simulink model "GREEN_CARM_DARM"  (Simulink 9.0)
settings: Solver=ode45  StartTime=0.0  StopTime=10.0  RelTol=1e-3  AbsTol=1e-6
values from neighbouring files (symbols this model uses):
  Actuator = [1,1/2;1,-1/2]    [run_NBGREEN_CARM_DARM.m]
  Changing_unit1 = c/L/532e-9    (= 187839885965)    [run_NBGREEN_CARM_DARM.m]
  CMRR_arm = 1    [run_NBGREEN_CARM_DARM.m]
  Noise = containers.Map    [run_NBGREEN_CARM_DARM.m]
  Sensing = [1,0;0,-1]    [run_NBGREEN_CARM_DARM.m]
  TransImp = containers.Map    [run_NBGREEN_CARM_DARM.m]
  use_AOM = 1    [run_NBGREEN_CARM_DARM.m]
  VertCoup = 0.01    [run_NBGREEN_CARM_DARM.m]
undefined symbols (not defined in the file or in its folder): Act, Cav, CavOpgain, CMS_SW_IMC, dt, myzpk, Suspension, SW
libraries: cstblocks x42, NbLibrary x35, mnNb_Lib x5
CloseFcn:
  | ;slview('closediagram',bdroot);
settings Model: SuppressorTable=22 serialization::archive 11 0 6 0 0 0 0 0  Creator=controls  LastModifiedBy=miyo  ExtModeTrigMode=oneshot  ExtModeArmWhenConnect=off
settings DataIOCC: SignalLoggingSaveFormat=ModelDataLogs
settings OptimizationCC: BlockReduction=off  BooleanDataType=off  DefaultParameterBehavior=Inlined  BufferReuse=off
settings DebuggingCC: SaveWithParameterizedLinksMsg=none  SignalResolutionControl=TryResolveAllWithWarning  MultiTaskDSMMsg=warning  MultiTaskCondExecSysMsg=none  StateNameClashWarn=warning  InitInArrayFormatMsg=none
settings HardwareCC: TargetUnknown=on
settings RTWCC: TemplateMakefile=grt_unix.tmf
settings GRTTargetCC: GeneratePreprocessorConditionals=Disable all  CombineOutputUpdateFcns=off  GRTInterface=on
settings ConfigComp: CovSFcnEnable=off

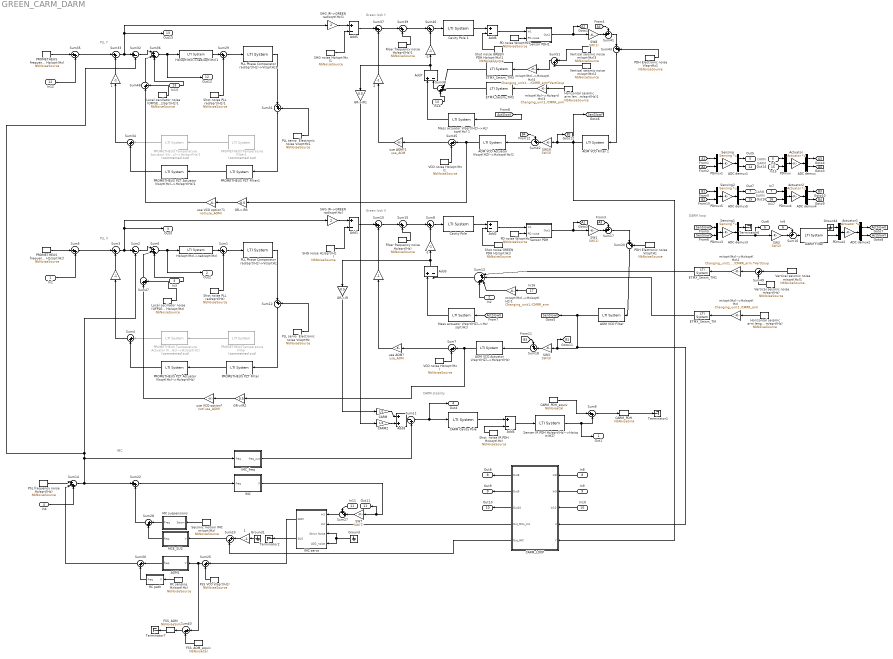
== system GREEN_CARM_DARM ==
  note: PLL X
  note: Green lock X
  note: IMC
  note: CARM stablity
  note: PLL Y
  note: Green lock Y
  note: CARM
  note: DARM
  note: CARM
  note: DARM
  note: DARM loop
  In1 : Inport
  In2 : Inport  Port=2
  In3 : Inport  Port=3
  In4 : Inport  Port=4
  In5 : Inport  Port=5
  In6 : Inport  Port=6
  In7 : Inport  Port=7
  In8 : Inport  Port=8
  In9 : Inport  Port=9
  In10 : Inport  Port=10
  In11 : Inport  Port=11
  In12 : Inport  Port=12
  In13 : Inport  Port=13
  In14 : Inport  Port=14
  In15 : Inport  Port=15
  In17 : Inport  Port=16
  In16 : Inport  Port=17
  " " : Gain  Gain=-1
  "  " : Gain  Gain=-1
  "  1" : Gain  Gain=-1
  " -1" : Gain  Gain=-1
  " -2" : Gain  Gain=-1
  " 1" : Gain  Gain=-1
  " 2" : Gain  Gain=-1
   GR->IR{,1..3} (4 alike) : Gain  Gain=0.5
  ADC demux{,1..5} (6 alike) : Demux  Outputs=2
  AOM VCO Actuator V/sqrt(HZ)-->Hz/sqrt(Hz) : cstblocks/LTI System  sys=Act_AOM_X  IC=[]
  AOM VCO Actuator V/sqrt(HZ)-->Hz/sqrt(Hz)1 : cstblocks/LTI System  sys=Act_AOM_Y  IC=[]
  "AOM VCO Filter " : cstblocks/LTI System  sys=Filt_GR1  IC=[]
  AOM VCO Filter 1 : cstblocks/LTI System  sys=Filt_GR1  IC=[]
  AOM1 : Subsystem
  Actuator : Gain  Gain=Actuator  Multiplication=Matrix(K*u)
  Actuator1 : Gain  Gain=Actuator  Multiplication=Matrix(K*u)
  Actuator2 : Gain  Gain=Actuator  Multiplication=Matrix(K*u)
  Add{1..7} (7 alike) : Sum  Inputs=+-
  Add8 : Sum
  CARM : Gain  Gain=1/2
  CARM Cavity Pole : cstblocks/LTI System  sys=CARM_Cavity_Pole  IC=[]
  CARM2 : Gain  Gain=1/2
  CARM_LOOP : Subsystem
  CARM_PDH : NbLibrary/NbNoiseSink  Tag=NbNoiseSink  dof='CARM'  asd=''  chan=''
      settings: AttributesFormatString=%<Tag>
  CARM_PDH_equiv : NbLibrary/NbNoiseCal  Tag=NbNoiseCal  dof='CARM'  unit='Frequency noise [Hz/rtHz]'
      settings: AttributesFormatString=%<Tag>
  "Cavity Pole " : cstblocks/LTI System  sys=Cavity_Pole  IC=[]
  Cavity Pole 1 : cstblocks/LTI System  sys=Cavity_Pole  IC=[]
  "DARM Filter " : cstblocks/LTI System  sys=Filt_darm  IC=[]
  ETMX_Seism_TM : cstblocks/LTI System  Description=FlexTf: Susp('ETMX_Seism_TM')  sys=1  IC=[]
      settings: AttributesFormatString=%<Description>
  ETMX_Seism_TM1 : cstblocks/LTI System  Description=FlexTf: Susp('ETMX_Seism_Vert')  sys=1  IC=[]
      settings: AttributesFormatString=%<Description>
  ETMX_Seism_TM2 : cstblocks/LTI System  Description=FlexTf: Susp('ETMX_Seism_TM')  sys=1  IC=[]
      settings: AttributesFormatString=%<Description>
  ETMX_Seism_TM3 : cstblocks/LTI System  Description=FlexTf: Susp('ETMX_Seism_Vert')  sys=1  IC=[]
      settings: AttributesFormatString=%<Description>
  FSS VCO V/sqrt(Hz) : NbLibrary/NbNoiseSource  Tag=NbNoiseSource  asd=Noise('act_AOM')  chan=''  groupNest=1  group='IR noise'  subgroup=''  subsubgroup=''  subsubsubgroup=''
      settings: AttributesFormatString=%<Tag>
  FSS_AOM : NbLibrary/NbNoiseSink  Tag=NbNoiseSink  dof='FSS_AOM'  asd=''  chan=''
      settings: AttributesFormatString=%<Tag>
  FSS_AOM_equiv : NbLibrary/NbNoiseCal  Tag=NbNoiseCal  dof='FSS_AOM'  unit='Feedback signal [V/rtHz]'
      settings: AttributesFormatString=%<Tag>
  Fiber frequency noise Hz/sqrt(Hz) : NbLibrary/NbNoiseSource  Tag=NbNoiseSource  asd=Noise('Fiber')  chan=''  groupNest=1  group='Green noise'  subgroup=''  subsubgroup=''  subsubsubgroup=''
      settings: AttributesFormatString=%<Tag>
  Fiber frequency noise Hz/sqrt(Hz)1 : NbLibrary/NbNoiseSource  Tag=NbNoiseSource  asd=Noise('Fiber')  chan=''  groupNest=1  group='Green noise'  subgroup=''  subsubgroup=''  subsubsubgroup=''
      settings: AttributesFormatString=%<Tag>
  Ground : Ground
  Ground1 : Ground
  Ground4 : Ground
  Horizontal seismic arm length m/sqrt(Hz) : NbLibrary/NbNoiseSource  Tag=NbNoiseSource  asd=Noise('Seismic arm length')  chan=''  groupNest=1  group='Seismic noise'  subgroup=''  subsubgroup=''  subsubsubgroup=''
      settings: AttributesFormatString=%<Tag>
  Horizontal seismic arm length m/sqrt(Hz)1 : NbLibrary/NbNoiseSource  Tag=NbNoiseSource  asd=Noise('Seismic arm length')  chan=''  groupNest=1  group='Seismic noise'  subgroup=''  subsubgroup=''  subsubsubgroup=''
      settings: AttributesFormatString=%<Tag>
  Hz/sqrt(Hz)->rad/sqrt(Hz) : cstblocks/LTI System  sys=Changing_unit  IC=[]
  Hz/sqrt(Hz)->rad/sqrt(Hz)1 : cstblocks/LTI System  sys=Changing_unit  IC=[]
  IMC : Subsystem
  IMC servo : Subsystem
  IMC_freq : Subsystem
  Local oscillator noise (OFFSET) Hz/sqrt(Hz) : NbLibrary/NbNoiseSource  Tag=NbNoiseSource  asd=Noise('LO noise')  chan=''  groupNest=1  group='PLL noise'  subgroup=''  subsubgroup=''  subsubsubgroup=''
      settings: AttributesFormatString=%<Tag>
  Local oscillator noise (OFFSET) Hz/sqrt(Hz)1 : NbLibrary/NbNoiseSource  Tag=NbNoiseSource  asd=Noise('LO noise')  chan=''  groupNest=1  group='PLL noise'  subgroup=''  subsubgroup=''  subsubsubgroup=''
      settings: AttributesFormatString=%<Tag>
  MC suspensions : Subsystem
  MCE_SUS : Subsystem
  "Mass actuator V/sqrt(HZ)-->Hz/sqrt(Hz) " : cstblocks/LTI System  sys=Act_mass  IC=[]
  Mass actuator V/sqrt(HZ)-->Hz/sqrt(Hz) 1 : cstblocks/LTI System  sys=Act_mass  IC=[]
  PD noise W/sqrtHz : NbLibrary/NbNoiseSource  Tag=NbNoiseSource  asd=Noise('PD noise PDH')  chan=''  groupNest=1  group='Green noise'  subgroup=''  subsubgroup=''  subsubsubgroup=''
      settings: AttributesFormatString=%<Tag>
  PD noise W/sqrtHz1 : NbLibrary/NbNoiseSource  Tag=NbNoiseSource  asd=Noise('PD noise PDH')  chan=''  groupNest=1  group='Green noise'  subgroup=''  subsubgroup=''  subsubsubgroup=''
      settings: AttributesFormatString=%<Tag>
  PDH Electronic noise V/sqrtHz : NbLibrary/NbNoiseSource  Tag=NbNoiseSource  asd=Noise('Electronic noise PDH')  chan=''  groupNest=1  group='Green noise'  subgroup=''  subsubgroup=''  subsubsubgroup=''
      settings: AttributesFormatString=%<Tag>
  PDH Electronic noise V/sqrtHz1 : NbLibrary/NbNoiseSource  Tag=NbNoiseSource  asd=Noise('Electronic noise PDH')  chan=''  groupNest=1  group='Green noise'  subgroup=''  subsubgroup=''  subsubsubgroup=''
      settings: AttributesFormatString=%<Tag>
  PDmux{,1..5} (6 alike) : Mux  Inputs=2
  PLL Phase Comparator rad/sqrt(Hz)->V/sqrtHz : cstblocks/LTI System  sys=Sen  IC=[]
  PLL Phase Comparator rad/sqrt(Hz)->V/sqrtHz1 : cstblocks/LTI System  sys=Sen  IC=[]
  PLL servo  Electronic noise V/sqrtHz : NbLibrary/NbNoiseSource  Tag=NbNoiseSource  asd=Noise('Electronic noise PLL')  chan=''  groupNest=1  group='PLL noise'  subgroup=''  subsubgroup=''  subsubsubgroup=''
      settings: AttributesFormatString=%<Tag>
  PLL servo  Electronic noise V/sqrtHz1 : NbLibrary/NbNoiseSource  Tag=NbNoiseSource  asd=Noise('Electronic noise PLL')  chan=''  groupNest=1  group='PLL noise'  subgroup=''  subsubgroup=''  subsubsubgroup=''
      settings: AttributesFormatString=%<Tag>
  PROMETHEUS PZT Actuator V/sqrt(Hz)-->Hz/sqrt(Hz) : cstblocks/LTI System  sys=Act_PZT  IC=[]
  PROMETHEUS PZT Actuator V/sqrt(Hz)-->Hz/sqrt(Hz)1 : cstblocks/LTI System  sys=Act_PZT  IC=[]
  PROMETHEUS PZT Filter : cstblocks/LTI System  sys=Filt_PZT  IC=[]
  PROMETHEUS PZT Filter1 : cstblocks/LTI System  sys=Filt_PZT  IC=[]
  PROMETHEUS Temperature Actuator V/sqrt(Hz)-->Hz/sqrt(Hz) : cstblocks/LTI System  Commented=on  sys=Act_Temp  IC=[]
  PROMETHEUS Temperature Actuator V/sqrt(Hz)-->Hz/sqrt(Hz)1 : cstblocks/LTI System  Commented=on  sys=Act_Temp  IC=[]
  PROMETHEUS frequency noise X Hz/sqrt(Hz) : NbLibrary/NbNoiseSource  Tag=NbNoiseSource  asd=Noise('Prometheus freq noise')  chan=''  groupNest=1  group='PLL noise'  subgroup=''  subsubgroup=''  subsubsubgroup=''
      settings: AttributesFormatString=%<Tag>
  PROMETHEUS frequency noise Y Hz/sqrt(Hz) : NbLibrary/NbNoiseSource  Tag=NbNoiseSource  asd=Noise('Prometheus freq noise')  chan=''  groupNest=1  group='PLL noise'  subgroup=''  subsubgroup=''  subsubsubgroup=''
      settings: AttributesFormatString=%<Tag>
  PROMETHEUSTemperature Filter : cstblocks/LTI System  Commented=on  sys=Filt_Temp  IC=[]
  PROMETHEUSTemperature Filter1 : cstblocks/LTI System  Commented=on  sys=Filt_Temp  IC=[]
  PSL frequency noise Hz/sqrt(Hz) : NbLibrary/NbNoiseSource  Tag=NbNoiseSource  asd=Noise('PSL freq noise')*0  chan=''  groupNest=1  group='IR noise'  subgroup=''  subsubgroup=''  subsubsubgroup=''
      settings: AttributesFormatString=%<Tag>
  RC path : Subsystem
  RC sensing Hz/sqrt(Hz) : NbLibrary/NbNoiseSource  Tag=NbNoiseSource  asd=Noise('sensor_RefCav')  chan=''  groupNest=1  group='IR noise'  subgroup=''  subsubgroup=''  subsubsubgroup=''
      settings: AttributesFormatString=%<Tag>
  SHG IR-->GREEN rad/sqrt(Hz) : Gain  Gain=2
  SHG IR-->GREEN rad/sqrt(Hz)1 : Gain  Gain=2
  SHG noise Hz/sqrt(Hz) : NbLibrary/NbNoiseSource  Tag=NbNoiseSource  asd=Noise('SHG')  chan=''  groupNest=1  group='Green noise'  subgroup=''  subsubgroup=''  subsubsubgroup=''
      settings: AttributesFormatString=%<Tag>
  SHG noise Hz/sqrt(Hz)1 : NbLibrary/NbNoiseSource  Tag=NbNoiseSource  asd=Noise('SHG')  chan=''  groupNest=1  group='Green noise'  subgroup=''  subsubgroup=''  subsubsubgroup=''
      settings: AttributesFormatString=%<Tag>
  SW1 : Gain  Gain=SW(1)
  SW10 : Gain  Gain=SW(3)
  SW2 : Gain  Gain=SW(2)
  SW3 : Gain  Gain=SW(3)
  SW7 : Gain  Gain=SW(7)
  SW8 : Gain  Gain=SW(1)
  Seismic motion IMC m/sqrt(Hz) : NbLibrary/NbNoiseSource  Tag=NbNoiseSource  asd=Noise('seismic_IMC')  chan=''  groupNest=1  group='IR noise'  subgroup=''  subsubgroup=''  subsubsubgroup=''
      settings: AttributesFormatString=%<Tag>
  Senser IR PDH Hz/sqrt(Hz)-->Hz/sqrt(HZ) : cstblocks/LTI System  sys=Sen_2  IC=[]
  Sensing : Gain  Gain=Sensing  Multiplication=Matrix(K*u)
  Sensing1 : Gain  Gain=Sensing  Multiplication=Matrix(K*u)
  Sensing2 : Gain  Gain=Sensing  Multiplication=Matrix(K*u)
  Sensor PDH : Subsystem
  Sensor PDH1 : Subsystem
  Shot  noise IR PDH Hz/sqrt(Hz) : NbLibrary/NbNoiseSource  Tag=NbNoiseSource  asd=Noise('Shot noise IR')  chan=''  groupNest=1  group='IR noise'  subgroup=''  subsubgroup=''  subsubsubgroup=''
      settings: AttributesFormatString=%<Tag>
  Shot noise GREEN PDH Hz/sqrt(Hz) : NbLibrary/NbNoiseSource  Tag=NbNoiseSource  asd=Noise('Shot noise green')  chan=''  groupNest=1  group='Green noise'  subgroup=''  subsubgroup=''  subsubsubgroup=''
      settings: AttributesFormatString=%<Tag>
  Shot noise GREEN PDH Hz/sqrt(Hz)1 : NbLibrary/NbNoiseSource  Tag=NbNoiseSource  asd=Noise('Shot noise green')  chan=''  groupNest=1  group='Green noise'  subgroup=''  subsubgroup=''  subsubsubgroup=''
      settings: AttributesFormatString=%<Tag>
  Shot noise PLL rad/sqrt(Hz) : NbLibrary/NbNoiseSource  Tag=NbNoiseSource  asd=Noise('Shot noise PLL')  chan=''  groupNest=1  group='PLL noise'  subgroup=''  subsubgroup=''  subsubsubgroup=''
      settings: AttributesFormatString=%<Tag>
  Shot noise PLL rad/sqrt(Hz)1 : NbLibrary/NbNoiseSource  Tag=NbNoiseSource  asd=Noise('Shot noise PLL')  chan=''  groupNest=1  group='PLL noise'  subgroup=''  subsubgroup=''  subsubsubgroup=''
      settings: AttributesFormatString=%<Tag>
  Sum{1,3..5,7..10,12,15,20,22..23,25,28..31,33..35,37,39..40,43,45..49,51} (31 alike) : Sum  Inputs=|++
  Sum11 : Sum  Inputs=|-+
  Sum13 : Sum  Inputs=|++++
  Sum14 : Sum  Inputs=|+-+
  Sum{16..18,27,41..42} (6 alike) : Sum  Inputs=++|
  Sum2 : Sum  Inputs=|+-
  Sum32 : Sum  Inputs=|+-
  Sum36 : Sum  Inputs=|+++
  Sum38 : Sum  Inputs=|+++
  Sum6 : Sum  Inputs=|+++
  Terminator{1..2,6..7} (4 alike) : Terminator
  VCO noise Hz/sqrt(Hz) : NbLibrary/NbNoiseSource  Tag=NbNoiseSource  asd=Noise('VCO noise')  chan=''  groupNest=1  group='Green noise'  subgroup=''  subsubgroup=''  subsubsubgroup=''
      settings: AttributesFormatString=%<Tag>
  VCO noise Hz/sqrt(Hz)1 : NbLibrary/NbNoiseSource  Tag=NbNoiseSource  asd=Noise('VCO noise')  chan=''  groupNest=1  group='Green noise'  subgroup=''  subsubgroup=''  subsubsubgroup=''
      settings: AttributesFormatString=%<Tag>
  Vertical seismic noise m/sqrt(Hz){,1..3} (4 alike) : NbLibrary/NbNoiseSource  Tag=NbNoiseSource  asd=Noise('Seismic test mass')  chan=''  groupNest=1  group='Seismic noise'  subgroup=''  subsubgroup=''  subsubsubgroup=''
      settings: AttributesFormatString=%<Tag>
  m/sqrt(Hz)-->Hz/sqrt(Hz) : Gain  Gain=Changing_unit1./CMRR_arm
  m/sqrt(Hz)-->Hz/sqrt(Hz)1 : Gain  Gain=Changing_unit1./CMRR_arm
  m/sqrt(Hz)-->Hz/sqrt(Hz)2 : Gain  Gain=Changing_unit1./CMRR_arm.*VertCoup
  m/sqrt(Hz)-->Hz/sqrt(Hz)3 : Gain  Gain=Changing_unit1./CMRR_arm
  m/sqrt(Hz)-->Hz/sqrt(Hz)4 : Gain  Gain=Changing_unit1./CMRR_arm*VertCoup
  use AOM? : Gain  Gain=use_AOM
  use AOM?1 : Gain  Gain=use_AOM
  use VCO option? : Gain  Gain=not(use_AOM)
  use VCO option?1 : Gain  Gain=not(use_AOM)
  Out1 : Outport
  Out2 : Outport  Port=2
  Out3 : Outport  Port=3
  Out4 : Outport  Port=4
  Out5 : Outport  Port=5
  Out6 : Outport  Port=6
  Out7 : Outport  Port=7
  Out8 : Outport  Port=8
  Out9 : Outport  Port=9
  Out10 : Outport  Port=10
  Out11 : Outport  Port=11
  Out12 : Outport  Port=12
  Out13 : Outport  Port=13
  Out14 : Outport  Port=14
  Out16 : Outport  Port=15
  tag scope: A1=global, A2=global, A3=global, A4=global, ActSlowX=global, ActSlowY=global, B1=global, B2=global, B3=global, B4=global, SenSlowX=global, SenSlowY=global
  wires:
  Sum4/1 -> "  "/1
  Local oscillator noise (OFFSET) Hz/sqrt(Hz)/1 -> Sum47/2
  Sum3/1 -> SHG IR-->GREEN rad/sqrt(Hz)/1, Out3/1, Sum2/1
  PROMETHEUSTemperature Filter/1 -> PROMETHEUS Temperature Actuator V/sqrt(Hz)-->Hz/sqrt(Hz)/1
  PROMETHEUS Temperature Actuator V/sqrt(Hz)-->Hz/sqrt(Hz)/1 -> Sum4/1
  Shot noise PLL rad/sqrt(Hz)/1 -> Sum1/2
  Sum9/1 -> CARM_PDH/1
  CARM_PDH_equiv/1 -> Sum9/1
  CARM_PDH/1 -> Terminator1/1
  Add1/1 -> Sum10/1
  VCO noise Hz/sqrt(Hz)/1 -> Sum7/2
  " "/1 -> Sum10/2
  SHG IR-->GREEN rad/sqrt(Hz)/1 -> Add1/1
  SHG noise Hz/sqrt(Hz)/1 -> Add1/2
  Add2/1 -> Sensor PDH/1(In1)
  Shot noise GREEN PDH Hz/sqrt(Hz)/1 -> Add2/2
  Add3/1 -> " -1"/1, " GR->IR"/1
  Shot  noise IR PDH Hz/sqrt(Hz)/1 -> Add4/2
  Senser IR PDH Hz/sqrt(Hz)-->Hz/sqrt(HZ)/1 -> Sum9/2, Out1/1
  PROMETHEUS frequency noise X Hz/sqrt(Hz)/1 -> Sum5/1
  Sum5/1 -> Sum3/1
  In1/1 -> Sum5/2
  PLL servo  Electronic noise V/sqrtHz/1 -> Sum12/2
  "  "/1 -> Sum3/2
  In2/1 -> Sum13/4
  ADC demux2/1 -> [ActSlowX]
  "Mass actuator V/sqrt(HZ)-->Hz/sqrt(Hz) "/1 -> Add3/1
  "Cavity Pole "/1 -> Add2/1
  Sum8/1 -> "Cavity Pole "/1
  Sum7/1 -> use AOM?/1
  AOM VCO Actuator V/sqrt(HZ)-->Hz/sqrt(Hz)/1 -> " GR->IR2"/1, Sum7/1
  Sum12/1 -> PROMETHEUS PZT Filter/1
  PROMETHEUS PZT Filter/1 -> PROMETHEUS PZT Actuator V/sqrt(Hz)-->Hz/sqrt(Hz)/1
  PROMETHEUS PZT Actuator V/sqrt(Hz)-->Hz/sqrt(Hz)/1 -> Sum4/2
  Sum1/1 -> PLL Phase Comparator rad/sqrt(Hz)->V/sqrtHz/1
  PLL Phase Comparator rad/sqrt(Hz)->V/sqrtHz/1 -> Sum12/1
  Hz/sqrt(Hz)->rad/sqrt(Hz)/1 -> Sum1/1
  PSL frequency noise Hz/sqrt(Hz)/1 -> Sum14/1
  In3/1 -> Sum6/3
  Sum2/1 -> Sum6/1
  Sum6/1 -> Out2/1, Hz/sqrt(Hz)->rad/sqrt(Hz)/1
  In4/1 -> Sum14/3
  Sum11/1 -> Out4/1, CARM Cavity Pole/1
  Sum10/1 -> Sum15/1
  Sum15/1 -> Sum8/1
  Fiber frequency noise Hz/sqrt(Hz)/1 -> Sum15/2
  " -1"/1 -> Sum8/2
  SW1/1 -> Sum17/2
  Sum17/1 -> Sum20/1
  [A3] -> Sum17/1
  Sensor PDH/1(Out1) -> [A1], SW1/1
  SW2/1 -> Sum16/2
  Sum16/1 -> "DARM Filter "/1
  In6/1 -> Sum16/1
  SW3/1 -> Sum18/2
  Sum18/1 -> AOM VCO Actuator V/sqrt(HZ)-->Hz/sqrt(Hz)/1
  [B3] -> Sum18/1
  CARM Cavity Pole/1 -> Add4/1
  Add4/1 -> Senser IR PDH Hz/sqrt(Hz)-->Hz/sqrt(HZ)/1
  PDH Electronic noise V/sqrtHz/1 -> Sum20/2
  Sum22/1 -> IMC/1(freq)
  Sum23/1 -> MCE_SUS/1(V)
  IMC_freq/1(freq_out) -> Sum11/2
  Ground/1 -> IMC servo/4(ADC_noise), IMC servo/3(Servo Noise)
  IMC servo/2("SUS ") -> Terminator2/1
  " 1"/1 -> Sum23/1
  Ground1/1 -> " 1"/1
  Sum28/1 -> Sum22/2
  FSS VCO V/sqrt(Hz)/1 -> Sum25/2
  SW7/1 -> Sum27/2
  Sum27/1 -> IMC servo/1(In1)
  In11/1 -> Sum27/1
  IMC/1(V) -> Out11/1, SW7/1
  MCE_SUS/1(freq) -> Sum28/2
  MC suspensions/1(Freq) -> Sum28/1
  Seismic motion IMC m/sqrt(Hz)/1 -> MC suspensions/1(Seism)
  Sum30/1 -> Sum14/2
  Sum25/1 -> AOM1/1(V), Sum40/1
  AOM1/1(freq) -> Sum30/1
  RC sensing Hz/sqrt(Hz)/1 -> RC path/1(V)
  RC path/1(freq) -> Sum30/2
  Sum13/1 -> Add3/2
  m/sqrt(Hz)-->Hz/sqrt(Hz)/1 -> ETMX_Seism_TM/1
  ETMX_Seism_TM/1 -> Sum13/2
  PD noise W/sqrtHz/1 -> Sensor PDH/2(PD noise)
  Sum34/1 -> "  1"/1
  Sum48/1 -> Sum36/2
  Sum14/1 -> Sum22/1, Sum32/2, Sum2/2, IMC_freq/1(freq)
  Sum33/1 -> SHG IR-->GREEN rad/sqrt(Hz)1/1, Out13/1, Sum32/1
  PROMETHEUSTemperature Filter1/1 -> PROMETHEUS Temperature Actuator V/sqrt(Hz)-->Hz/sqrt(Hz)1/1
  PROMETHEUS Temperature Actuator V/sqrt(Hz)-->Hz/sqrt(Hz)1/1 -> Sum34/1
  Shot noise PLL rad/sqrt(Hz)1/1 -> Sum29/2
  PROMETHEUS frequency noise Y Hz/sqrt(Hz)/1 -> Sum35/1
  Sum35/1 -> Sum33/1
  In12/1 -> Sum35/2
  PLL servo  Electronic noise V/sqrtHz1/1 -> Sum31/2
  "  1"/1 -> Sum33/2
  Sum31/1 -> PROMETHEUS PZT Filter1/1
  PROMETHEUS PZT Filter1/1 -> PROMETHEUS PZT Actuator V/sqrt(Hz)-->Hz/sqrt(Hz)1/1
  PROMETHEUS PZT Actuator V/sqrt(Hz)-->Hz/sqrt(Hz)1/1 -> Sum34/2
  Sum29/1 -> PLL Phase Comparator rad/sqrt(Hz)->V/sqrtHz1/1
  PLL Phase Comparator rad/sqrt(Hz)->V/sqrtHz1/1 -> Sum31/1
  Hz/sqrt(Hz)->rad/sqrt(Hz)1/1 -> Sum29/1
  In13/1 -> Sum36/3
  Sum32/1 -> Sum36/1
  Sum36/1 -> Out12/1, Hz/sqrt(Hz)->rad/sqrt(Hz)1/1
  Add5/1 -> Sum37/1
  VCO noise Hz/sqrt(Hz)1/1 -> Sum45/2
  " 2"/1 -> Sum37/2
  SHG IR-->GREEN rad/sqrt(Hz)1/1 -> Add5/1
  SHG noise Hz/sqrt(Hz)1/1 -> Add5/2
  Add6/1 -> Sensor PDH1/1(In1)
  Shot noise GREEN PDH Hz/sqrt(Hz)1/1 -> Add6/2
  Add7/1 -> " GR->IR1"/1, " -2"/1
  In14/1 -> Sum38/3
  ADC demux2/2 -> [ActSlowY]
  Mass actuator V/sqrt(HZ)-->Hz/sqrt(Hz) 1/1 -> Add7/1
  Cavity Pole 1/1 -> Add6/1
  Sum46/1 -> Cavity Pole 1/1
  Sum45/1 -> use AOM?1/1
  Sum37/1 -> Sum39/1
  Sum39/1 -> Sum46/1
  Fiber frequency noise Hz/sqrt(Hz)1/1 -> Sum39/2
  " -2"/1 -> Sum46/2
  SW8/1 -> Sum41/2
  Sum41/1 -> Sum43/1
  [A4] -> Sum41/1
  Sensor PDH1/1(Out1) -> [A2], SW8/1
  SW10/1 -> Sum42/2
  Sum42/1 -> AOM VCO Actuator V/sqrt(HZ)-->Hz/sqrt(Hz)1/1
  [B4] -> Sum42/1
  PDH Electronic noise V/sqrtHz1/1 -> Sum43/2
  Sum38/1 -> Add7/2
  PD noise W/sqrtHz1/1 -> Sensor PDH1/2(PD noise)
  " GR->IR1"/1 -> CARM2/1
  CARM/1 -> Add8/1
  CARM2/1 -> Add8/2
  Add8/1 -> Sum11/1
  " GR->IR"/1 -> CARM/1
  Actuator/1 -> ADC demux/1
  PDmux/1 -> Actuator/1
  PDmux1/1 -> Sensing/1
  Sensing/1 -> ADC demux1/1
  [A1] -> PDmux1/1
  [A2] -> PDmux1/2
  ADC demux/1 -> [A3]
  ADC demux/2 -> [A4]
  ADC demux1/1 -> Out5/1
  ADC demux1/2 -> Out14/1
  In15/1 -> PDmux/2
  In5/1 -> PDmux/1
  Actuator1/1 -> ADC demux2/1
  PDmux2/1 -> Actuator1/1
  PDmux3/1 -> Sensing1/1
  Sensing1/1 -> ADC demux3/1
  "AOM VCO Filter "/1 -> CARM_LOOP/4(X), [B1], SW3/1, [SenSlowX]
  ADC demux3/1 -> Terminator6/1
  ADC demux3/2 -> Out6/1, SW2/1
  "DARM Filter "/1 -> PDmux2/2
  Ground4/1 -> PDmux2/1
  [SenSlowX] -> PDmux3/1
  [SenSlowY] -> PDmux3/2
  [ActSlowY] -> Mass actuator V/sqrt(HZ)-->Hz/sqrt(Hz) 1/1
  [ActSlowX] -> "Mass actuator V/sqrt(HZ)-->Hz/sqrt(Hz) "/1
  Actuator2/1 -> ADC demux4/1
  PDmux4/1 -> Actuator2/1
  PDmux5/1 -> Sensing2/1
  Sensing2/1 -> ADC demux5/1
  [B1] -> PDmux5/1
  [B2] -> PDmux5/2
  ADC demux4/1 -> [B3]
  ADC demux4/2 -> [B4]
  ADC demux5/1 -> Out7/1
  ADC demux5/2 -> Out16/1
  In17/1 -> PDmux4/2
  In7/1 -> PDmux4/1
  Sum20/1 -> "AOM VCO Filter "/1
  Sum43/1 -> AOM VCO Filter 1/1
  IMC servo/1("AOM ") -> Sum25/1
  Sum40/1 -> FSS_AOM/1
  FSS_AOM_equiv/1 -> Sum40/2
  FSS_AOM/1 -> Terminator7/1
  Sum47/1 -> Sum6/2
  " GR->IR2"/1 -> use VCO option?/1
  use AOM?/1 -> " "/1
  use VCO option?/1 -> Sum47/1
  AOM VCO Actuator V/sqrt(HZ)-->Hz/sqrt(Hz)1/1 -> " GR->IR3"/1, Sum45/1
  " GR->IR3"/1 -> use VCO option?1/1
  use VCO option?1/1 -> Sum48/1
  use AOM?1/1 -> " 2"/1
  Local oscillator noise (OFFSET) Hz/sqrt(Hz)1/1 -> Sum48/2
  Vertical seismic noise m/sqrt(Hz)1/1 -> Sum49/1
  Vertical seismic noise m/sqrt(Hz)/1 -> Sum49/2
  Sum49/1 -> m/sqrt(Hz)-->Hz/sqrt(Hz)2/1
  m/sqrt(Hz)-->Hz/sqrt(Hz)2/1 -> ETMX_Seism_TM1/1
  ETMX_Seism_TM1/1 -> Sum13/1
  m/sqrt(Hz)-->Hz/sqrt(Hz)3/1 -> ETMX_Seism_TM2/1
  ETMX_Seism_TM2/1 -> Sum38/2
  Vertical seismic noise m/sqrt(Hz)3/1 -> Sum51/1
  Vertical seismic noise m/sqrt(Hz)2/1 -> Sum51/2
  Sum51/1 -> m/sqrt(Hz)-->Hz/sqrt(Hz)4/1
  m/sqrt(Hz)-->Hz/sqrt(Hz)4/1 -> ETMX_Seism_TM3/1
  ETMX_Seism_TM3/1 -> Sum38/1
  Horizontal seismic arm length m/sqrt(Hz)1/1 -> m/sqrt(Hz)-->Hz/sqrt(Hz)3/1
  In16/1 -> m/sqrt(Hz)-->Hz/sqrt(Hz)1/1
  m/sqrt(Hz)-->Hz/sqrt(Hz)1/1 -> Sum13/3
  Horizontal seismic arm length m/sqrt(Hz)/1 -> m/sqrt(Hz)-->Hz/sqrt(Hz)/1
  CARM_LOOP/5(Out_IMC) -> Sum23/2
  CARM_LOOP/3(Out10) -> Out10/1
  CARM_LOOP/1(Out8) -> Out8/1
  CARM_LOOP/2(Out9) -> Out9/1
  In8/1 -> CARM_LOOP/1(In8)
  In9/1 -> CARM_LOOP/2(In9)
  In10/1 -> CARM_LOOP/3(In10)
  AOM VCO Filter 1/1 -> CARM_LOOP/5(Y), [B2], SW10/1, [SenSlowY]
  CARM_LOOP/4(Out_MCL_In2) -> IMC servo/2(In2)

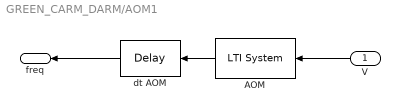
== system GREEN_CARM_DARM/AOM1 ==
  V : Inport
  "AOM " : cstblocks/LTI System  sys=Act('AOM')  IC=[]
  dt AOM : TransportDelay  DelayTime=dt('AOM')
  freq : Outport
  wires:
  "AOM "/1 -> dt AOM/1
  V/1 -> "AOM "/1
  dt AOM/1 -> freq/1

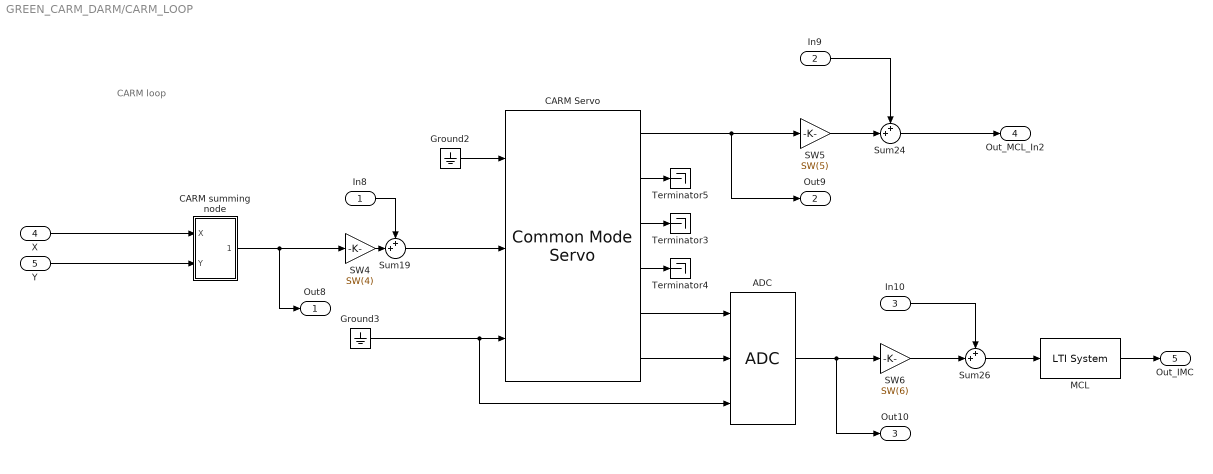
== system GREEN_CARM_DARM/CARM_LOOP ==
  note: CARM loop
  In8 : Inport
  In9 : Inport  Port=2
  In10 : Inport  Port=3
  X : Inport  Port=4
  Y : Inport  Port=5
  ADC : mnNb_Lib/RTS/ADC
      link override gain: Gain=2
  CARM Servo : mnNb_Lib/Servo/Common Mode Servo  CMS_Elec=CMS_Elec_CARM  CMS_SW=CMS_SW_CARM
  CARM summing node : Subsystem
  Ground2 : Ground
  Ground3 : Ground
  MCL : cstblocks/LTI System  sys=Filt_MCL  IC=[]
  SW4 : Gain  Gain=SW(4)
  SW5 : Gain  Gain=SW(5)
  SW6 : Gain  Gain=SW(6)
  Sum19 : Sum  Inputs=++|
  Sum24 : Sum  Inputs=++|
  Sum26 : Sum  Inputs=++|
  Terminator3 : Terminator
  Terminator4 : Terminator
  Terminator5 : Terminator
  Out8 : Outport
  Out9 : Outport  Port=2
  Out10 : Outport  Port=3
  Out_MCL_In2 : Outport  Port=4
  Out_IMC : Outport  Port=5
  wires:
  SW4/1 -> Sum19/2
  CARM summing node/1(Out1) -> Out8/1, SW4/1
  CARM Servo/4 -> Terminator4/1
  Sum19/1 -> CARM Servo/2
  CARM Servo/5 -> ADC/1
  ADC/1 -> SW6/1, Out10/1
  In9/1 -> Sum24/1
  CARM Servo/1 -> Out9/1, SW5/1
  In8/1 -> Sum19/1
  CARM Servo/6 -> ADC/2
  SW5/1 -> Sum24/2
  Ground2/1 -> CARM Servo/1
  CARM Servo/3 -> Terminator3/1
  Ground3/1 -> ADC/3, CARM Servo/3
  In10/1 -> Sum26/1
  SW6/1 -> Sum26/2
  CARM Servo/2 -> Terminator5/1
  Sum26/1 -> MCL/1
  MCL/1 -> Out_IMC/1
  X/1 -> CARM summing node/1(X)
  Y/1 -> CARM summing node/2(Y)
  Sum24/1 -> Out_MCL_In2/1

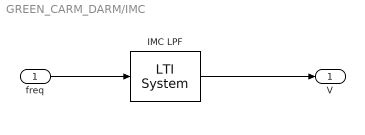
== system GREEN_CARM_DARM/IMC ==
  freq : Inport
  IMC LPF : cstblocks/LTI System  sys=CavOpgain('IMC')  IC=[]
  V : Outport
  wires:
  freq/1 -> IMC LPF/1
  IMC LPF/1 -> V/1

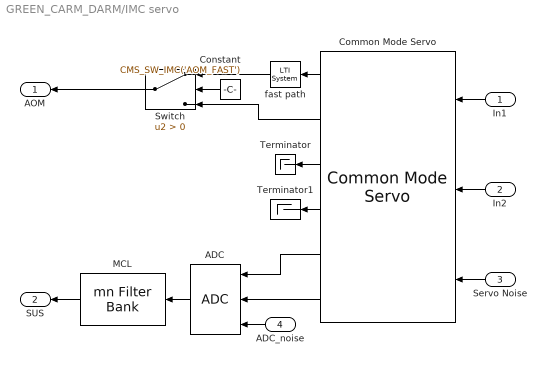
== system GREEN_CARM_DARM/IMC servo ==
  In1 : Inport
  In2 : Inport  Port=2
  Servo Noise : Inport  Port=3
  ADC_noise : Inport  Port=4
  ADC : mnNb_Lib/RTS/ADC
      link override gain: Gain=2
  Common Mode Servo : mnNb_Lib/Servo/Common Mode Servo  CMS_Elec=CMS_Elec  CMS_SW=CMS_SW_IMC
  Constant : Constant  Value=CMS_SW_IMC('AOM_FAST')
  MCL : mnNb_Lib/RTS/mn Filter Bank  Chan='K1:IMC-MCL_SERVO'  FB=FB  FB_SW=FB_SW_MCL
  Switch : Switch  Criteria=u2 > Threshold
  Terminator : Terminator
  Terminator1 : Terminator
  fast path : cstblocks/LTI System  sys=change_filter  IC=[]
  "AOM " : Outport
  "SUS " : Outport  Port=2
  wires:
  MCL/1 -> "SUS "/1
  ADC/1 -> MCL/1
  In1/1 -> Common Mode Servo/1
  ADC_noise/1 -> ADC/3
  Servo Noise/1 -> Common Mode Servo/3
  In2/1 -> Common Mode Servo/2
  Common Mode Servo/5 -> ADC/1
  Common Mode Servo/6 -> ADC/2
  Common Mode Servo/4 -> Terminator1/1
  Common Mode Servo/3 -> Terminator/1
  Constant/1 -> Switch/2
  Switch/1 -> "AOM "/1
  Common Mode Servo/1 -> fast path/1
  Common Mode Servo/2 -> Switch/3
  fast path/1 -> Switch/1

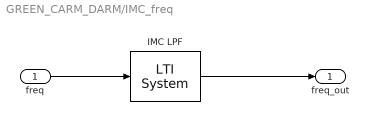
== system GREEN_CARM_DARM/IMC_freq ==
  freq : Inport
  IMC LPF : cstblocks/LTI System  sys=myzpk('zpk',[],[Cav('Cpole_IMC')],1)  IC=[]
  freq_out : Outport
  wires:
  freq/1 -> IMC LPF/1
  IMC LPF/1 -> freq_out/1

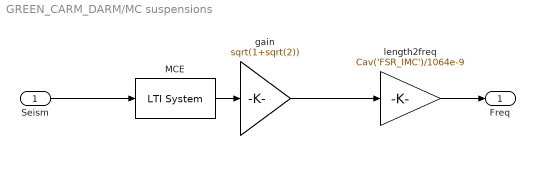
== system GREEN_CARM_DARM/MC suspensions ==
  Seism : Inport
  MCE : cstblocks/LTI System  sys=Suspension('MCE')  IC=[]
  gain : Gain  Gain=sqrt(1+sqrt(2))
  length2freq : Gain  Gain=Cav('FSR_IMC')/1064e-9
  Freq : Outport
  wires:
  Seism/1 -> MCE/1
  MCE/1 -> gain/1
  gain/1 -> length2freq/1
  length2freq/1 -> Freq/1

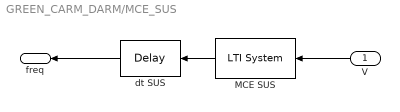
== system GREEN_CARM_DARM/MCE_SUS ==
  V : Inport
  MCE SUS : cstblocks/LTI System  sys=Act('MCEsus')  IC=[]
  dt SUS : TransportDelay  DelayTime=dt('MCEsus')
  freq : Outport
  wires:
  V/1 -> MCE SUS/1
  MCE SUS/1 -> dt SUS/1
  dt SUS/1 -> freq/1

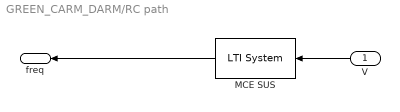
== system GREEN_CARM_DARM/RC path ==
  V : Inport
  MCE SUS : cstblocks/LTI System  sys=1/CavOpgain('RefCav')*myzpk('zpk',[],[1e6;1e6],1)  IC=[]
  freq : Outport
  wires:
  V/1 -> MCE SUS/1
  MCE SUS/1 -> freq/1

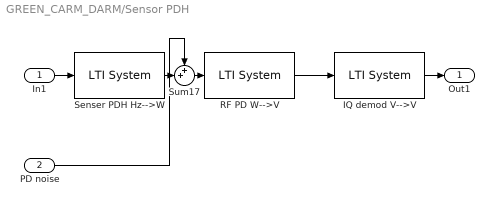
== system GREEN_CARM_DARM/Sensor PDH ==
  In1 : Inport
  PD noise : Inport  Port=2
  IQ demod V-->V : cstblocks/LTI System  sys=DeModGain  IC=[]
  RF PD W-->V : cstblocks/LTI System  sys=TransImp('green')  IC=[]
  Senser PDH Hz-->W : cstblocks/LTI System  sys=green_PDH  IC=[]
  Sum17 : Sum  Inputs=++|
  Out1 : Outport
  wires:
  RF PD W-->V/1 -> IQ demod V-->V/1
  In1/1 -> Senser PDH Hz-->W/1
  IQ demod V-->V/1 -> Out1/1
  Sum17/1 -> RF PD W-->V/1
  Senser PDH Hz-->W/1 -> Sum17/2
  PD noise/1 -> Sum17/1

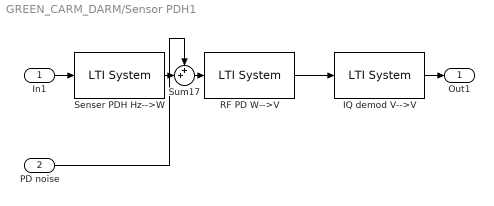
== system GREEN_CARM_DARM/Sensor PDH1 ==
  In1 : Inport
  PD noise : Inport  Port=2
  IQ demod V-->V : cstblocks/LTI System  sys=DeModGain  IC=[]
  RF PD W-->V : cstblocks/LTI System  sys=TransImp('green')  IC=[]
  Senser PDH Hz-->W : cstblocks/LTI System  sys=green_PDH  IC=[]
  Sum17 : Sum  Inputs=++|
  Out1 : Outport
  wires:
  RF PD W-->V/1 -> IQ demod V-->V/1
  In1/1 -> Senser PDH Hz-->W/1
  IQ demod V-->V/1 -> Out1/1
  Sum17/1 -> RF PD W-->V/1
  Senser PDH Hz-->W/1 -> Sum17/2
  PD noise/1 -> Sum17/1

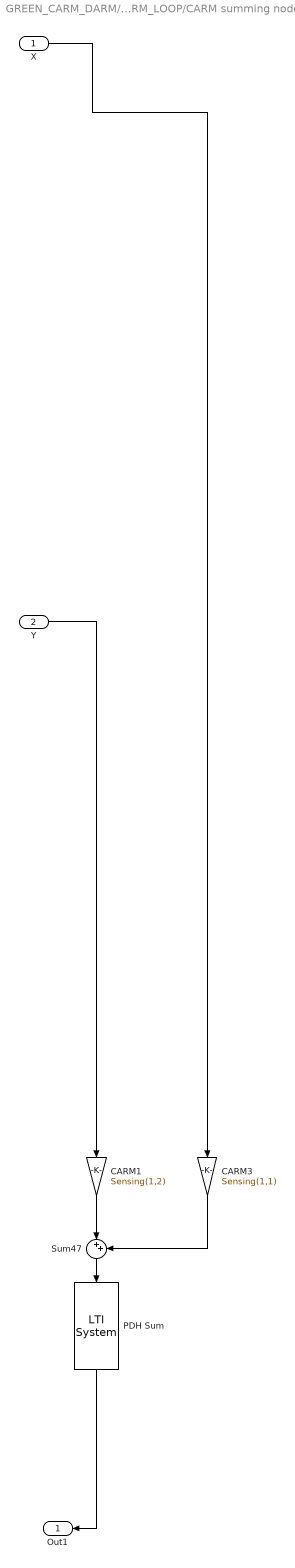
== system GREEN_CARM_DARM/CARM_LOOP/CARM summing node ==
  X : Inport
  Y : Inport  Port=2
  CARM1 : Gain  Gain=Sensing(1,2)
  CARM3 : Gain  Gain=Sensing(1,1)
  PDH Sum : cstblocks/LTI System  sys=Filt_sum  IC=[]
  Sum47 : Sum  Inputs=|++
  Out1 : Outport
  wires:
  CARM1/1 -> Sum47/1
  Y/1 -> CARM1/1
  X/1 -> CARM3/1
  Sum47/1 -> PDH Sum/1
  CARM3/1 -> Sum47/2
  PDH Sum/1 -> Out1/1
